simulink model "simulink_ICE2"  (R2023b)
settings: Solver=VariableStepAuto  StartTime=0.0  StopTime=10.0  RelTol=1e-3
values from neighbouring files (symbols this model uses):
  A = [0 1 ... (first row only)    [ICE.m]    (also in ICE2.m)
  B = [0 1 ... (first row only)    [ICE.m]    (also in ICE2.m = [0; 1])
  K = M / X    [ICE2.m]
settings Model: Creator=USER_55_LAPTOP  LastModifiedBy=USER_55_LAPTOP

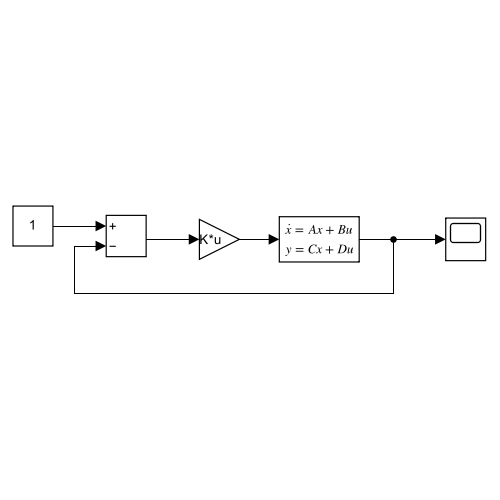
[thumbnail: Simulink's stored preview of the top-level diagram]
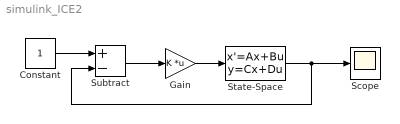
== system simulink_ICE2 ==
  Constant : Constant  OutMin=[0]  OutMax=[1]
  Gain : Gain  Gain=K  Multiplication=Matrix(K*u)
  Scope : Scope
  State-Space : StateSpace  A=A  B=B  C=[1 0; 1 0]  D=[0; 0]  InitialCondition=[0; 0]
  Subtract : Sum  Inputs=+-
  wires:
  State-Space/1 -> Subtract/2, Scope/1
  Gain/1 -> State-Space/1
  Subtract/1 -> Gain/1
  Constant/1 -> Subtract/1
